simulink model "car_speed_control_uart_test"  (R2024b)
settings: Solver=FixedStepAuto  StartTime=0.0  StopTime=300  FixedStep=0.5  RelTol=1e-3  EnableMultiTasking=on
libraries: arduinolib x2, simulink_extras x1
settings Model: ExtModeTrigDuration=2  Creator=USER  LastModifiedBy=USER
settings SolverCC: AutoInsertRateTranBlk=on
settings OptimizationCC: EnhancedBackFolding=on  PassReuseOutputArgsAs=Individual arguments  ZeroExternalMemoryAtStartup=off  ZeroInternalMemoryAtStartup=off  MaxStackSize=64  OptimizeBlockOrder=speed  DifferentSizesBufferReuse=on  OptimizationCustomize=off  EfficientTunableParamExpr=on
settings DebuggingCC: ParameterTunabilityLossMsg=error
settings HardwareCC: ProdBitPerInt=16  ProdBitPerPointer=16  ProdBitPerSizeT=16  ProdBitPerPtrDiffT=16  ProdLargestAtomicFloat=None  ProdWordSize=8  ProdHWDeviceType=Atmel->AVR
settings SFSimCC: MATLABDynamicMemAlloc=off
settings RTWCC: Description=Embedded Coder  SystemTargetFile=ert.tlc  HardwareBoard=Arduino Mega 2560  GenCodeOnly=on  TemplateMakefile=ert_default_tmf  Toolchain=Arduino AVR  BuildConfiguration=Faster Runs
settings CodeAppCC: ForceParamTrailComments=on  IgnoreCustomStorageClasses=off  OperatorAnnotations=on  SimulinkDataObjDesc=on  SFDataObjDesc=on  InsertBlockDesc=on
settings ERTTargetCC: SupportContinuousTime=on  SupportVariableSizeSignals=on  ExtModeTransport=3  ExtModeStaticAlloc=on  ExtModeAutomaticAllocSize=off  ExtModeStaticAllocSize=2048  ExtModeMexFile=ext_xcp  ExtModeIntrfLevel=Level2 - Open  InlinedParameterPlacement=Hierarchical

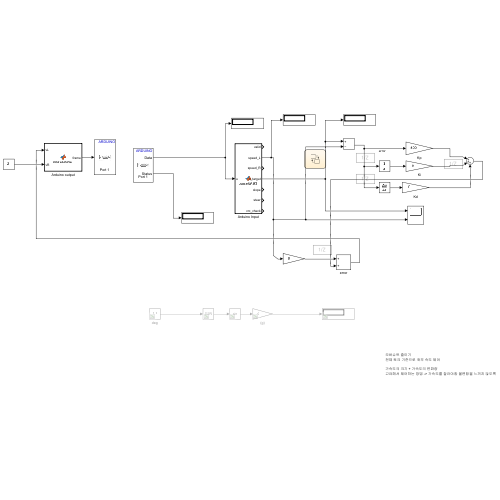
[thumbnail: Simulink's stored preview of the top-level diagram]
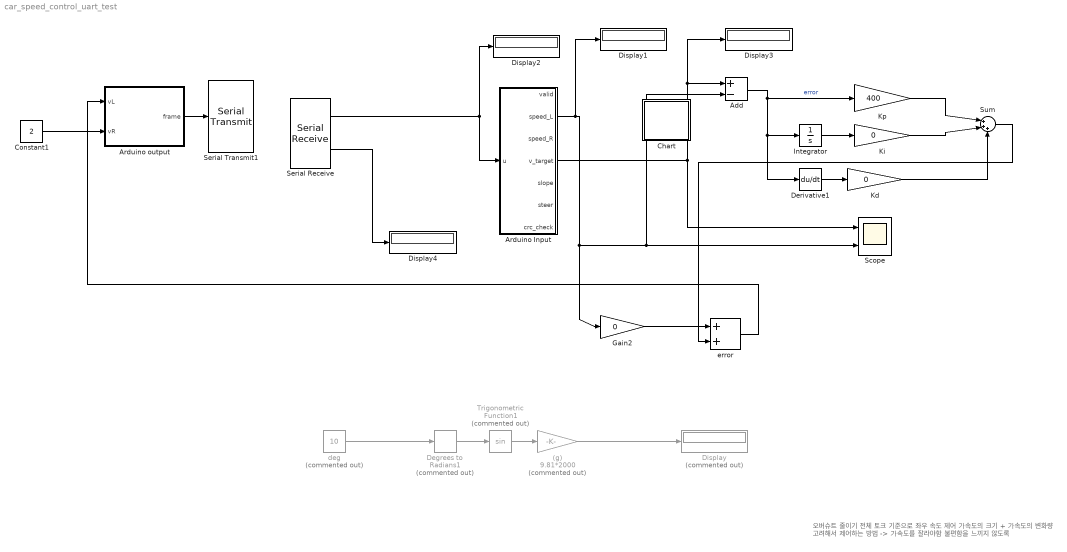
== system car_speed_control_uart_test ==
  note: 오버슈트 줄이기
      | 전체 토크 기준으로 좌우 속도 제어
      |
      | 가속도의 크기 + 가속도의 변화량
      | 고려해서 제어하는 방법 -> 가속도를 잘라야함 불편함을 느끼지 않도록
  (g) : Gain  Commented=on  Gain=9.81*2000
  Add : Sum  Inputs=+-
  Arduino Input : MATLAB Function  TreatAsAtomicUnit=on
  Arduino output : MATLAB Function  TreatAsAtomicUnit=on
  Chart : Stateflow chart  TreatAsAtomicUnit=on
  Constant1 : Constant  Value=2
  Degrees to Radians1 : simulink_extras/Transformations/Degrees to Radians  Commented=on
  Derivative1 : Derivative
  Display : Display  Commented=on
  Display{1..4} (4 alike) : Display
  Gain2 : Gain  Gain=0
  Integrator : Integrator
  Kd : Gain  Gain=0
  Ki : Gain  Gain=0
  Kp : Gain  Gain=400
  Scope : Scope  NumInputPorts=2
  Serial Receive : arduinolib/Serial Receive  portNumber=1  DataType=uint8  blockPlatform=ARDUINO  TimeOut=0  MaxDataLength=10  isARMArch=off  DataLengthOption=Length via dialog  Datalength=7  Header=[]  Terminator=[]  SampleTime=1  ShowOutStatus=on
      settings: SourceProductName=Common
  Serial Transmit1 : arduinolib/Serial Transmit  portNumber=1  sendmode=write  sendformat=Decimal  floatprecision=2  header=[]  terminator=[]  blockPlatform=ARDUINO
      settings: SourceProductName=Common
  Sum : Sum  Inputs=|+++
  Trigonometric Function1 : Trigonometry  Commented=on
  deg : Constant  Commented=on  Value=10
  error : Sum
  wires:
  Arduino Input/2(speed_L) -> Display1/1, Gain2/1, Add/2, Scope/2
  Arduino Input/4(v_target) -> Display3/1, Add/1, Scope/1
  Add/1 -> Derivative1/1, Integrator/1, Kp/1  "error"
  Gain2/1 -> error/1
  deg/1 -> Degrees to Radians1/1
  Degrees to Radians1/1 -> Trigonometric Function1/1
  Trigonometric Function1/1 -> (g)/1
  (g)/1 -> Display/1
  Integrator/1 -> Ki/1
  Derivative1/1 -> Kd/1
  Kp/1 -> Sum/1
  Ki/1 -> Sum/2
  Kd/1 -> Sum/3
  Sum/1 -> error/2
  Serial Receive/1 -> Arduino Input/1(u), Display2/1
  Arduino output/1(frame) -> Serial Transmit1/1
  Constant1/1 -> Arduino output/2(vR)
  Serial Receive/2 -> Display4/1
  error/1 -> Arduino output/1(vL)

== matlab function car_speed_control_uart_test/Arduino output ==
  data: vL input; frame output; vR input
function frame = makeFrame(vL, vR)
% 입력:
%   vL, vR : 좌/우 목표 속도 (실수, cm/s 단위)
% 출력:
%   frame : 7-byte UART 전송 프레임 (uint8 벡터)

    frame = zeros(7,1,'uint8');  % 7바이트 프레임

    % 1. Start Byte
    frame(1) = hex2dec('AA');

    % 2-3. 목표속도_L (정수 + 소수)
    frame(2) = uint8(floor(vL));                       % 정수부
    frame(3) = uint8(floor(mod(vL * 100, 100)));       % 소수부 (소수점 둘째 자리까지)

    % 4-5. 목표속도_R (정수 + 소수)
    frame(4) = uint8(floor(vR));                       % 정수부
    frame(5) = uint8(floor(mod(vR * 100, 100)));       % 소수부

    % 6. CRC: 256 - (sum of byte 1~5) % 256
    crc = mod(sum(double(frame(1:5))), 256);
    frame(6) = uint8(mod(256 - crc, 256));
    
    % 7. End Byte
    frame(7) = hex2dec('55');
end

== matlab function car_speed_control_uart_test/Arduino Input ==
  data: valid output; speed_L output; speed_R output; v_target output; u input; slope output; steer output; crc_check output
function [valid, speed_L, speed_R, v_target, slope, steer, crc_check] = parseUART(u)
% 입력: u [10x1 uint8]
% 출력:
%   valid     : 1이면 유효한 프레임
%   speed_L   : 왼쪽 속도 (double, cm/s)
%   speed_R   : 오른쪽 속도 (double, cm/s)
%   v_target  : 목표 속도 (uint8, cm/s)
%   slope     : 경사각 (uint8, degree)
%   steer     : 조향각 (int8, degree)
%   crc_check : CRC 검증 성공 여부 (1: OK, 0: fail)

% 기본값 초기화
valid = 0;
crc_check = 0;
speed_L = 0.0;
speed_R = 0.0;
v_target = 0;
slope = 0;
steer = 0;

% 프레임 유효성 확인
if length(u) == 10 && u(1) == hex2dec('AA') && u(10) == hex2dec('55')
    
    % CRC 검사
    sum_payload = sum(double(u(1:8)));
    crc = double(u(9));
    
    if mod(sum_payload + crc, 256) == 0
        crc_check = 1;
        valid = 1;
        
        % 속도 L = 정수 + 소수 / 100
        speed_L = double(u(2)) + double(u(3)) / 100;
        
        % 속도 R = 정수 + 소수 / 100
        speed_R = double(u(4)) + double(u(5)) / 100;
        
        % 목표 속도
        v_target = double(u(6));
        
        % 경사각
        slope = double(u(7));
        
        % 조향각 (signed 처리)
        steer = int8(u(8));
    end
end

== stateflow chart car_speed_control_uart_test/Chart ==
